simulink model "MAIN"  (R2023b)
settings: Solver=FixedStepDiscrete  StartTime=0.0  StopTime=inf  FixedStep=0.001  RelTol=1e-3  EnableMultiTasking=on
libraries: arduinolib x8, arduinosamdlib x1, arduinosensorlib x1
settings Model: ExtModeTrigDuration=2  Creator=NOA  LastModifiedBy=NOA
settings OptimizationCC: EnhancedBackFolding=on  PassReuseOutputArgsAs=Individual arguments  ZeroExternalMemoryAtStartup=off  ZeroInternalMemoryAtStartup=off  MaxStackSize=64  OptimizeBlockOrder=speed  DifferentSizesBufferReuse=on  OptimizationCustomize=off  EfficientTunableParamExpr=on
settings DebuggingCC: ParameterTunabilityLossMsg=error
settings HardwareCC: ProdBitPerInt=16  ProdBitPerPointer=16  ProdBitPerSizeT=16  ProdBitPerPtrDiffT=16  ProdLargestAtomicFloat=None  ProdWordSize=8  ProdHWDeviceType=Atmel->AVR  UseEmbeddedCoderFeatures=off  UseSimulinkCoderFeatures=off
settings SFSimCC: MATLABDynamicMemAlloc=off
settings RTWCC: Description=Embedded Coder  SystemTargetFile=ert.tlc  HardwareBoard=Arduino Uno  TemplateMakefile=ert_default_tmf  Toolchain=Arduino AVR  BuildConfiguration=Faster Runs
settings CodeAppCC: ForceParamTrailComments=on  IgnoreCustomStorageClasses=off  OperatorAnnotations=on  SimulinkDataObjDesc=on  SFDataObjDesc=on  MangleLength=10  InsertBlockDesc=on
settings ERTTargetCC: SupportContinuousTime=on  SupportNonInlinedSFcns=on  SupportVariableSizeSignals=on  ExtModeTransport=3  ExtModeStaticAlloc=on  ExtModeAutomaticAllocSize=off  ExtModeStaticAllocSize=250  ExtModeMexFile=ext_xcp  ExtModeIntrfLevel=Level2 - Open

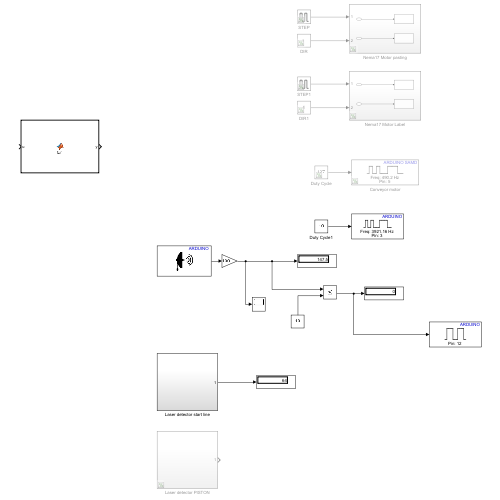
[thumbnail: Simulink's stored preview of the top-level diagram]
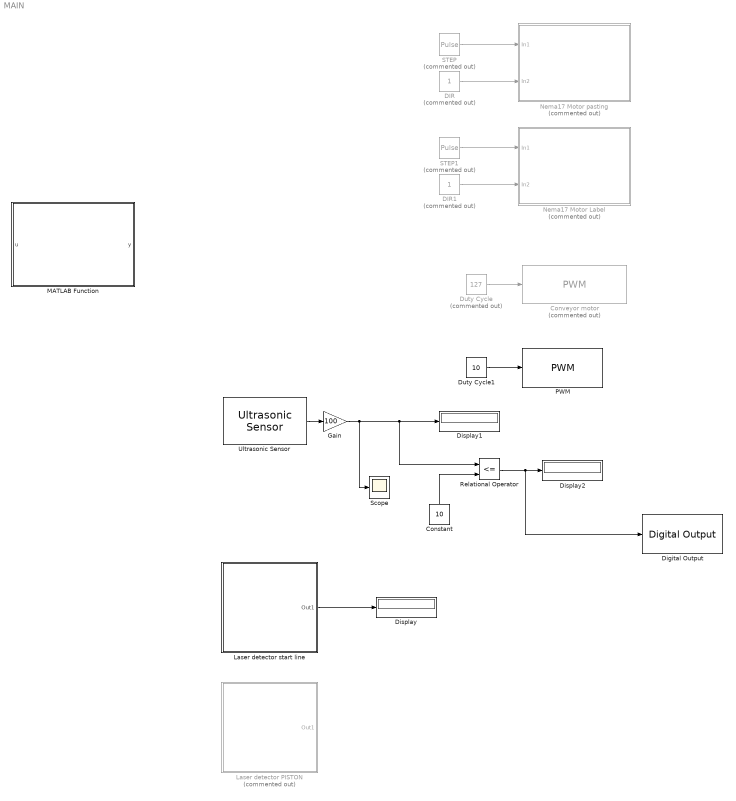
== system MAIN ==
  Constant : Constant  Value=10
  Conveyor motor : arduinosamdlib/PWM  Commented=on  pinNumber=5  desiredFrequency=490.2  achievableFrequency=490.2  wavegenMode=Dual-slope, interrupt/event at TOP (DSTOP)  EnableCompareMatchInterrupt=off  EnableOverflowInterrupt=on  InvertOutputPolarity=off
      settings: LibrarySourceBlock=arduinolib/PWM
  DIR : Constant  Commented=on
  DIR1 : Constant  Commented=on
  Digital Output : arduinolib/Digital Output  pinNumber=12  Direction=output  blockPlatform=arduino
  Display : Display
  Display1 : Display
  Display2 : Display
  Duty Cycle : Constant  Commented=on  Value=127
  Duty Cycle1 : Constant  Value=10
  Gain : Gain  Gain=100
  Laser detector PISTON : Subsystem  Commented=on
  Laser detector start line : Subsystem
  MATLAB Function : MATLAB Function  TreatAsAtomicUnit=on
  Nema17 Motor Label : Subsystem  Commented=on
  Nema17 Motor pasting : Subsystem  Commented=on
  PWM : arduinolib/PWM  pinNumber=3  frequencyType=Specify  desiredFrequency=3921.16  achievableFrequency=3921.16
  Relational Operator : RelationalOperator  Operator=<=  OutDataTypeStr=boolean  RndMeth=Simplest  InputSameDT=off
  STEP : DiscretePulseGenerator  Commented=on  PulseType=Time based  Period=0.002  PulseWidth=50
  STEP1 : DiscretePulseGenerator  Commented=on  PulseType=Time based  Period=0.002  PulseWidth=50
  Scope : Scope
  Ultrasonic Sensor : arduinosensorlib/Ultrasonic Sensor  NumSignalPins=2  TrigPin=4  EchoPin=5  SignalPin=3  SampleTime_=0.01  blockPlatform=ARDUINO
  wires:
  STEP/1 -> Nema17 Motor pasting/1(In1)
  DIR/1 -> Nema17 Motor pasting/2(In2)
  STEP1/1 -> Nema17 Motor Label/1(In1)
  DIR1/1 -> Nema17 Motor Label/2(In2)
  Duty Cycle/1 -> Conveyor motor/1
  Duty Cycle1/1 -> PWM/1
  Laser detector start line/1(Out1) -> Display/1
  Ultrasonic Sensor/1 -> Gain/1
  Gain/1 -> Scope/1, Relational Operator/1, Display1/1
  Constant/1 -> Relational Operator/2
  Relational Operator/1 -> Digital Output/1, Display2/1

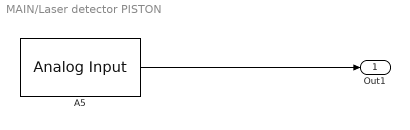
== system MAIN/Laser detector PISTON ==
  A5 : arduinolib/Analog Input  pinNumber=4  ReadResultsOnly=off  ConversionTriggerSource=Software  ExternalTriggerType=uint32( 0 )  OutputDataType=uint16  EnableConversionCompleteNotify=off  EnableOuputStatus=off  SampleTime=-1  blockPlatform=arduino
  Out1 : Outport
  wires:
  A5/1 -> Out1/1

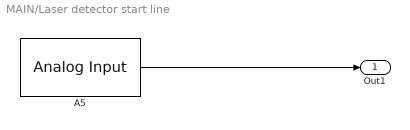
== system MAIN/Laser detector start line ==
  A5 : arduinolib/Analog Input  pinNumber=5  ReadResultsOnly=off  ConversionTriggerSource=Software  ExternalTriggerType=uint32( 0 )  OutputDataType=uint16  EnableConversionCompleteNotify=off  EnableOuputStatus=off  SampleTime=-1  blockPlatform=arduino
  Out1 : Outport
  wires:
  A5/1 -> Out1/1

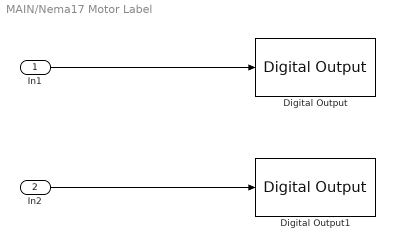
== system MAIN/Nema17 Motor Label ==
  In1 : Inport
  In2 : Inport  Port=2
  Digital Output : arduinolib/Digital Output  pinNumber=12  Direction=output  blockPlatform=arduino
  Digital Output1 : arduinolib/Digital Output  pinNumber=13  Direction=output  blockPlatform=arduino
  wires:
  In1/1 -> Digital Output/1
  In2/1 -> Digital Output1/1

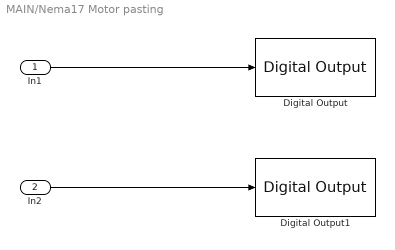
== system MAIN/Nema17 Motor pasting ==
  In1 : Inport
  In2 : Inport  Port=2
  Digital Output : arduinolib/Digital Output  pinNumber=12  Direction=output  blockPlatform=arduino
  Digital Output1 : arduinolib/Digital Output  pinNumber=13  Direction=output  blockPlatform=arduino
  wires:
  In1/1 -> Digital Output/1
  In2/1 -> Digital Output1/1

== matlab function MAIN/MATLAB Function ==
  data: u input; y output
function y = fcn(u)

y = u;
